simulink model "quad_full_control"  (R2024b)
settings: Solver=ode1  StartTime=0.0  StopTime=inf  FixedStep=0.01  RelTol=1e-3
libraries: slpidlib x4, uavutilslib x1
settings Model: Creator=ercu  LastModifiedBy=ercu

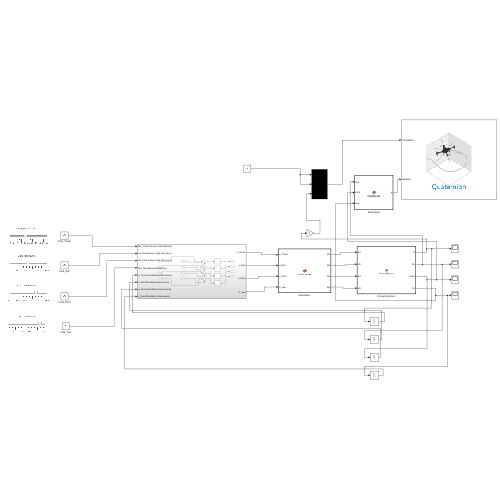
[thumbnail: Simulink's stored preview of the top-level diagram]
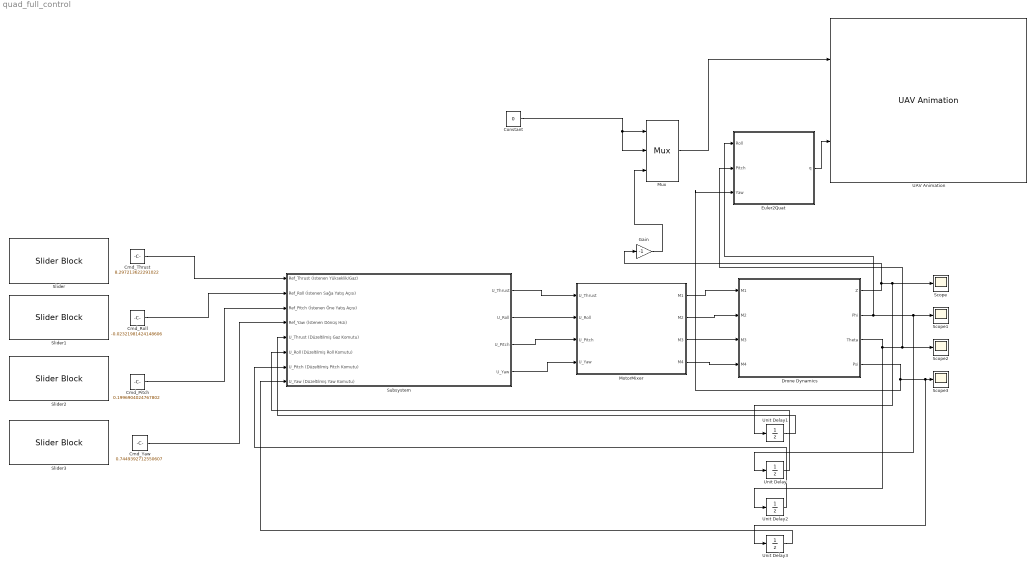
== system quad_full_control ==
  Cmd_Pitch : Constant  Value=0.1996904024767802
  Cmd_Roll : Constant  Value=-0.02321981424148606
  Cmd_Thrust : Constant  Value=8.297213622291022
  Cmd_Yaw : Constant  Value=0.7449392712550607
  Constant : Constant  Value=0
  Drone Dynamics : MATLAB Function  TreatAsAtomicUnit=on
  Euler2Quat : MATLAB Function  TreatAsAtomicUnit=on
  Gain : Gain  Gain=-1
  MotorMixer : MATLAB Function  TreatAsAtomicUnit=on
  Mux : Mux  Inputs=3
  Scope{,1..3} (4 alike) : Scope
  Slider : SliderBlock  ScaleMax=20
  Slider1 : SliderBlock  ScaleMin=-0.5  ScaleMax=0.5
  Slider2 : SliderBlock  ScaleMin=-0.5  ScaleMax=0.5
  Slider3 : SliderBlock  ScaleMin=-1  ScaleMax=1
  Subsystem : Subsystem
  UAV Animation : uavutilslib/UAV Animation  NumUAV=1  DynamicUAVConfig=off  UAVType=Multirotor  UAVSize=1  UAVColor=[1 0 0]  UAVTrajectoryAlpha=1  InertialZDirection=Down  RotationFormat=Quaternion  DrawMarkers=off  SampleTime=-1
  Unit Delay{,1..3} (4 alike) : UnitDelay  SampleTime=-1  HasFrameUpgradeWarning=on
  wires:
  MotorMixer/1(M1) -> Drone Dynamics/1(M1)
  MotorMixer/2(M2) -> Drone Dynamics/2(M2)
  MotorMixer/3(M3) -> Drone Dynamics/3(M3)
  MotorMixer/4(M4) -> Drone Dynamics/4(M4)
  Subsystem/1(U_Thrust) -> MotorMixer/1(U_Thrust)
  Subsystem/2(U_Roll) -> MotorMixer/2(U_Roll)
  Subsystem/3(U_Pitch) -> MotorMixer/3(U_Pitch)
  Subsystem/4(U_Yaw) -> MotorMixer/4(U_Yaw)
  Cmd_Roll/1 -> Subsystem/2(Ref_Roll (İstenen Sağa Yatış Açısı))
  Cmd_Pitch/1 -> Subsystem/3(Ref_Pitch (İstenen Öne Yatış Açısı))
  Cmd_Yaw/1 -> Subsystem/4(Ref_Yaw (İstenen Dönüş Hızı))
  Drone Dynamics/1(Z) -> Gain/1, Unit Delay1/1, Scope/1
  Drone Dynamics/2(Phi) -> Euler2Quat/1(Roll), Unit Delay/1, Scope1/1
  Drone Dynamics/3(Theta) -> Unit Delay2/1, Euler2Quat/2(Pitch), Scope2/1
  Drone Dynamics/4(Psi) -> Euler2Quat/3(Yaw), Unit Delay3/1, Scope3/1
  Unit Delay1/1 -> Subsystem/5(U_Thrust (Düzeltilmiş Gaz Komutu))
  Unit Delay/1 -> Subsystem/6(U_Roll (Düzeltilmiş Roll Komutu))
  Unit Delay2/1 -> Subsystem/7(U_Pitch (Düzeltilmiş Pitch Komutu))
  Unit Delay3/1 -> Subsystem/8(U_Yaw (Düzeltilmiş Yaw Komutu))
  Constant/1 -> Mux/2, Mux/1
  Mux/1 -> UAV Animation/1
  Euler2Quat/1(q) -> UAV Animation/2
  Cmd_Thrust/1 -> Subsystem/1(Ref_Thrust (İstenen Yükseklik/Gaz))
  Gain/1 -> Mux/3

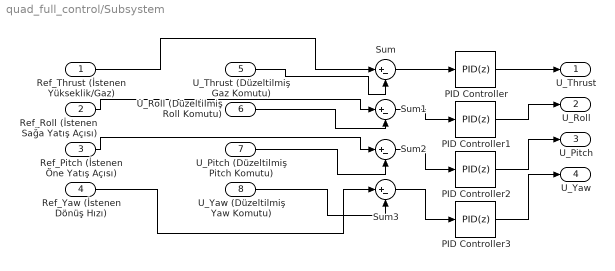
== system quad_full_control/Subsystem ==
  Ref_Thrust (İstenen Yükseklik/Gaz) : Inport
  Ref_Roll (İstenen Sağa Yatış Açısı) : Inport  Port=2
  Ref_Pitch (İstenen Öne Yatış Açısı) : Inport  Port=3
  Ref_Yaw (İstenen Dönüş Hızı) : Inport  Port=4
  U_Thrust (Düzeltilmiş Gaz Komutu) : Inport  Port=5
  U_Roll (Düzeltilmiş Roll Komutu) : Inport  Port=6
  U_Pitch (Düzeltilmiş Pitch Komutu) : Inport  Port=7
  U_Yaw (Düzeltilmiş Yaw Komutu) : Inport  Port=8
  PID Controller : slpidlib/PID Controller  Controller=PID  Form=Parallel  TimeDomain=Discrete-time  UseExternalTs=off  SampleTime=0.01  IntegratorMethod=Forward Euler  FilterMethod=Forward Euler  ControllerParametersSource=internal  P=3  I=1.5  UseKiTs=off  D=2.5  UseExternalDerivativeSource=off  N=100  UseFilter=on  TunerSelectOption=Transfer Function Based (PID Tuner App)  InitialConditionSource=internal  InitialConditionForIntegrator=0  InitialConditionForFilter=0  DifferentiatorICPrevScaledInput=0  ExternalReset=none  TrackingMode=off  Kt=1  LimitOutput=off  SatLimitsSource=internal  UpperSaturationLimit=inf  LowerSaturationLimit=-inf  LinearizeAsGain=on  AntiWindupMode=none  Kb=1  LimitIntegrator=off  UpperIntegratorSaturationLimit=inf  LowerIntegratorSaturationLimit=-inf  POutMin=[]  POutMax=[]  IOutMin=[]  IOutMax=[]  DOutMin=[]  DOutMax=[]  NOutMin=[]  NOutMax=[]  SumOutMin=[]  SumOutMax=[]  SaturationOutMin=[]  SaturationOutMax=[]  PParamMin=[]  PParamMax=[]  IParamMin=[]  IParamMax=[]  DParamMin=[]  DParamMax=[]  NParamMin=[]  NParamMax=[]  KbParamMin=[]  KbParamMax=[]  KtParamMin=[]  KtParamMax=[]  KbOutMin=[]  KbOutMax=[]  KtOutMin=[]  KtOutMax=[]  IntegratorOutMin=[]  IntegratorOutMax=[]  FilterOutMin=[]  FilterOutMax=[]  SumI1OutMin=[]  SumI1OutMax=[]  SumI2OutMin=[]  SumI2OutMax=[]  SumI3OutMin=[]  SumI3OutMax=[]  SumI4OutMin=[]  SumI4OutMax=[]  SumDOutMin=[]  SumDOutMax=[]  DifferentiatorOutMin=[]  DifferentiatorOutMax=[]  FilterDiffOutCoefMin=[]  FilterDiffOutCoefMax=[]  ReciprocalOutMin=[]  ReciprocalOutMax=[]  SumDenOutMin=[]  SumDenOutMax=[]  SumNumOutMin=[]  SumNumOutMax=[]  DivideOutMin=[]  DivideOutMax=[]  UdiffTsProdOutMin=[]  UdiffTsProdOutMax=[]  NTsProdOutMin=[]  NTsProdOutMax=[]  UintegralTsProdOutMin=[]  UintegralTsProdOutMax=[]  UngainTsProdOutMin=[]  UngainTsProdOutMax=[]  ClampingZeroOutDataTypeStr=Inherit: Inherit via back propagation  ClampingZeroOutMin=[]  ClampingZeroOutMax=[]  FilterDenConstantOutDataTypeStr=Inherit: Inherit via back propagation  FilterDenConstantOutMin=[]  FilterDenConstantOutMax=[]  PCopyOutDataTypeStr=Inherit: Inherit via back propagation  PCopyOutMin=[]  PCopyOutMax=[]  NCopyOutDataTypeStr=Inherit: Inherit via back propagation  NCopyOutMin=[]  NCopyOutMax=[]  IntegratorContinuousStateAttributes=''  IntegratorStateMustResolveToSignalObject=off  IntegratorRTWStateStorageClass=Auto  FilterContinuousStateAttributes=''  FilterStateMustResolveToSignalObject=off  FilterRTWStateStorageClass=Auto  ParallelPVariant=InternalParameters  IdealPVariant=Disabled  IVariant=InternalParameters  DVariant=InternalParameters  IntegratorVariant=Discrete  SatVariant=Disabled  AWVariant=Passthrough  PCopyVariant=Disabled  TRVariant=Disabled  FdbkBlocksVariant=Forward  IdealPFdbkVariant=Disabled  SatFdbkVariant=Disabled  DerivativeFilterVariant=ForwardEulerFilter  NVariant=InternalParameters  NCopyVariant=Disabled  FilterICVariant=InternalICsFilter  IntegratorICVariant=InternalICs  ExternalResetVariant=Disabled  TRSumVariant=Passthrough  SumFdbkVariant=Disabled  SumVariant=Sum_PID  TsampFilterVariant=InternalTs  TsampNgainVariant=Passthrough  TsampIntegralVariant=Disabled_SignalSpec  ExternalSaturationOutDataTypeStr=Inherit: Same as second input  DerivativeSourceVariant=ErrorSignal  PreIntVariant=InternalPreInt
  PID Controller1 : slpidlib/PID Controller  Controller=PID  Form=Parallel  TimeDomain=Discrete-time  UseExternalTs=off  SampleTime=0.01  IntegratorMethod=Forward Euler  FilterMethod=Forward Euler  ControllerParametersSource=internal  P=2  I=0  UseKiTs=off  D=0.5  UseExternalDerivativeSource=off  N=100  UseFilter=on  TunerSelectOption=Transfer Function Based (PID Tuner App)  InitialConditionSource=internal  InitialConditionForIntegrator=0  InitialConditionForFilter=0  DifferentiatorICPrevScaledInput=0  ExternalReset=none  TrackingMode=off  Kt=1  LimitOutput=off  SatLimitsSource=internal  UpperSaturationLimit=inf  LowerSaturationLimit=-inf  LinearizeAsGain=on  AntiWindupMode=none  Kb=1  LimitIntegrator=off  UpperIntegratorSaturationLimit=inf  LowerIntegratorSaturationLimit=-inf  POutMin=[]  POutMax=[]  IOutMin=[]  IOutMax=[]  DOutMin=[]  DOutMax=[]  NOutMin=[]  NOutMax=[]  SumOutMin=[]  SumOutMax=[]  SaturationOutMin=[]  SaturationOutMax=[]  PParamMin=[]  PParamMax=[]  IParamMin=[]  IParamMax=[]  DParamMin=[]  DParamMax=[]  NParamMin=[]  NParamMax=[]  KbParamMin=[]  KbParamMax=[]  KtParamMin=[]  KtParamMax=[]  KbOutMin=[]  KbOutMax=[]  KtOutMin=[]  KtOutMax=[]  IntegratorOutMin=[]  IntegratorOutMax=[]  FilterOutMin=[]  FilterOutMax=[]  SumI1OutMin=[]  SumI1OutMax=[]  SumI2OutMin=[]  SumI2OutMax=[]  SumI3OutMin=[]  SumI3OutMax=[]  SumI4OutMin=[]  SumI4OutMax=[]  SumDOutMin=[]  SumDOutMax=[]  DifferentiatorOutMin=[]  DifferentiatorOutMax=[]  FilterDiffOutCoefMin=[]  FilterDiffOutCoefMax=[]  ReciprocalOutMin=[]  ReciprocalOutMax=[]  SumDenOutMin=[]  SumDenOutMax=[]  SumNumOutMin=[]  SumNumOutMax=[]  DivideOutMin=[]  DivideOutMax=[]  UdiffTsProdOutMin=[]  UdiffTsProdOutMax=[]  NTsProdOutMin=[]  NTsProdOutMax=[]  UintegralTsProdOutMin=[]  UintegralTsProdOutMax=[]  UngainTsProdOutMin=[]  UngainTsProdOutMax=[]  ClampingZeroOutDataTypeStr=Inherit: Inherit via back propagation  ClampingZeroOutMin=[]  ClampingZeroOutMax=[]  FilterDenConstantOutDataTypeStr=Inherit: Inherit via back propagation  FilterDenConstantOutMin=[]  FilterDenConstantOutMax=[]  PCopyOutDataTypeStr=Inherit: Inherit via back propagation  PCopyOutMin=[]  PCopyOutMax=[]  NCopyOutDataTypeStr=Inherit: Inherit via back propagation  NCopyOutMin=[]  NCopyOutMax=[]  IntegratorContinuousStateAttributes=''  IntegratorStateMustResolveToSignalObject=off  IntegratorRTWStateStorageClass=Auto  FilterContinuousStateAttributes=''  FilterStateMustResolveToSignalObject=off  FilterRTWStateStorageClass=Auto  ParallelPVariant=InternalParameters  IdealPVariant=Disabled  IVariant=InternalParameters  DVariant=InternalParameters  IntegratorVariant=Discrete  SatVariant=Disabled  AWVariant=Passthrough  PCopyVariant=Disabled  TRVariant=Disabled  FdbkBlocksVariant=Forward  IdealPFdbkVariant=Disabled  SatFdbkVariant=Disabled  DerivativeFilterVariant=ForwardEulerFilter  NVariant=InternalParameters  NCopyVariant=Disabled  FilterICVariant=InternalICsFilter  IntegratorICVariant=InternalICs  ExternalResetVariant=Disabled  TRSumVariant=Passthrough  SumFdbkVariant=Disabled  SumVariant=Sum_PID  TsampFilterVariant=InternalTs  TsampNgainVariant=Passthrough  TsampIntegralVariant=Disabled_SignalSpec  ExternalSaturationOutDataTypeStr=Inherit: Same as second input  DerivativeSourceVariant=ErrorSignal  PreIntVariant=InternalPreInt
  PID Controller2 : slpidlib/PID Controller  Controller=PID  Form=Parallel  TimeDomain=Discrete-time  UseExternalTs=off  SampleTime=0.01  IntegratorMethod=Forward Euler  FilterMethod=Forward Euler  ControllerParametersSource=internal  P=2  I=0  UseKiTs=off  D=0.5  UseExternalDerivativeSource=off  N=100  UseFilter=on  TunerSelectOption=Transfer Function Based (PID Tuner App)  InitialConditionSource=internal  InitialConditionForIntegrator=0  InitialConditionForFilter=0  DifferentiatorICPrevScaledInput=0  ExternalReset=none  TrackingMode=off  Kt=1  LimitOutput=off  SatLimitsSource=internal  UpperSaturationLimit=inf  LowerSaturationLimit=-inf  LinearizeAsGain=on  AntiWindupMode=none  Kb=1  LimitIntegrator=off  UpperIntegratorSaturationLimit=inf  LowerIntegratorSaturationLimit=-inf  POutMin=[]  POutMax=[]  IOutMin=[]  IOutMax=[]  DOutMin=[]  DOutMax=[]  NOutMin=[]  NOutMax=[]  SumOutMin=[]  SumOutMax=[]  SaturationOutMin=[]  SaturationOutMax=[]  PParamMin=[]  PParamMax=[]  IParamMin=[]  IParamMax=[]  DParamMin=[]  DParamMax=[]  NParamMin=[]  NParamMax=[]  KbParamMin=[]  KbParamMax=[]  KtParamMin=[]  KtParamMax=[]  KbOutMin=[]  KbOutMax=[]  KtOutMin=[]  KtOutMax=[]  IntegratorOutMin=[]  IntegratorOutMax=[]  FilterOutMin=[]  FilterOutMax=[]  SumI1OutMin=[]  SumI1OutMax=[]  SumI2OutMin=[]  SumI2OutMax=[]  SumI3OutMin=[]  SumI3OutMax=[]  SumI4OutMin=[]  SumI4OutMax=[]  SumDOutMin=[]  SumDOutMax=[]  DifferentiatorOutMin=[]  DifferentiatorOutMax=[]  FilterDiffOutCoefMin=[]  FilterDiffOutCoefMax=[]  ReciprocalOutMin=[]  ReciprocalOutMax=[]  SumDenOutMin=[]  SumDenOutMax=[]  SumNumOutMin=[]  SumNumOutMax=[]  DivideOutMin=[]  DivideOutMax=[]  UdiffTsProdOutMin=[]  UdiffTsProdOutMax=[]  NTsProdOutMin=[]  NTsProdOutMax=[]  UintegralTsProdOutMin=[]  UintegralTsProdOutMax=[]  UngainTsProdOutMin=[]  UngainTsProdOutMax=[]  ClampingZeroOutDataTypeStr=Inherit: Inherit via back propagation  ClampingZeroOutMin=[]  ClampingZeroOutMax=[]  FilterDenConstantOutDataTypeStr=Inherit: Inherit via back propagation  FilterDenConstantOutMin=[]  FilterDenConstantOutMax=[]  PCopyOutDataTypeStr=Inherit: Inherit via back propagation  PCopyOutMin=[]  PCopyOutMax=[]  NCopyOutDataTypeStr=Inherit: Inherit via back propagation  NCopyOutMin=[]  NCopyOutMax=[]  IntegratorContinuousStateAttributes=''  IntegratorStateMustResolveToSignalObject=off  IntegratorRTWStateStorageClass=Auto  FilterContinuousStateAttributes=''  FilterStateMustResolveToSignalObject=off  FilterRTWStateStorageClass=Auto  ParallelPVariant=InternalParameters  IdealPVariant=Disabled  IVariant=InternalParameters  DVariant=InternalParameters  IntegratorVariant=Discrete  SatVariant=Disabled  AWVariant=Passthrough  PCopyVariant=Disabled  TRVariant=Disabled  FdbkBlocksVariant=Forward  IdealPFdbkVariant=Disabled  SatFdbkVariant=Disabled  DerivativeFilterVariant=ForwardEulerFilter  NVariant=InternalParameters  NCopyVariant=Disabled  FilterICVariant=InternalICsFilter  IntegratorICVariant=InternalICs  ExternalResetVariant=Disabled  TRSumVariant=Passthrough  SumFdbkVariant=Disabled  SumVariant=Sum_PID  TsampFilterVariant=InternalTs  TsampNgainVariant=Passthrough  TsampIntegralVariant=Disabled_SignalSpec  ExternalSaturationOutDataTypeStr=Inherit: Same as second input  DerivativeSourceVariant=ErrorSignal  PreIntVariant=InternalPreInt
  PID Controller3 : slpidlib/PID Controller  Controller=PID  Form=Parallel  TimeDomain=Discrete-time  UseExternalTs=off  SampleTime=0.01  IntegratorMethod=Forward Euler  FilterMethod=Forward Euler  ControllerParametersSource=internal  P=4  I=0.5  UseKiTs=off  D=0  UseExternalDerivativeSource=off  N=100  UseFilter=on  TunerSelectOption=Transfer Function Based (PID Tuner App)  InitialConditionSource=internal  InitialConditionForIntegrator=0  InitialConditionForFilter=0  DifferentiatorICPrevScaledInput=0  ExternalReset=none  TrackingMode=off  Kt=1  LimitOutput=off  SatLimitsSource=internal  UpperSaturationLimit=inf  LowerSaturationLimit=-inf  LinearizeAsGain=on  AntiWindupMode=none  Kb=1  LimitIntegrator=off  UpperIntegratorSaturationLimit=inf  LowerIntegratorSaturationLimit=-inf  POutMin=[]  POutMax=[]  IOutMin=[]  IOutMax=[]  DOutMin=[]  DOutMax=[]  NOutMin=[]  NOutMax=[]  SumOutMin=[]  SumOutMax=[]  SaturationOutMin=[]  SaturationOutMax=[]  PParamMin=[]  PParamMax=[]  IParamMin=[]  IParamMax=[]  DParamMin=[]  DParamMax=[]  NParamMin=[]  NParamMax=[]  KbParamMin=[]  KbParamMax=[]  KtParamMin=[]  KtParamMax=[]  KbOutMin=[]  KbOutMax=[]  KtOutMin=[]  KtOutMax=[]  IntegratorOutMin=[]  IntegratorOutMax=[]  FilterOutMin=[]  FilterOutMax=[]  SumI1OutMin=[]  SumI1OutMax=[]  SumI2OutMin=[]  SumI2OutMax=[]  SumI3OutMin=[]  SumI3OutMax=[]  SumI4OutMin=[]  SumI4OutMax=[]  SumDOutMin=[]  SumDOutMax=[]  DifferentiatorOutMin=[]  DifferentiatorOutMax=[]  FilterDiffOutCoefMin=[]  FilterDiffOutCoefMax=[]  ReciprocalOutMin=[]  ReciprocalOutMax=[]  SumDenOutMin=[]  SumDenOutMax=[]  SumNumOutMin=[]  SumNumOutMax=[]  DivideOutMin=[]  DivideOutMax=[]  UdiffTsProdOutMin=[]  UdiffTsProdOutMax=[]  NTsProdOutMin=[]  NTsProdOutMax=[]  UintegralTsProdOutMin=[]  UintegralTsProdOutMax=[]  UngainTsProdOutMin=[]  UngainTsProdOutMax=[]  ClampingZeroOutDataTypeStr=Inherit: Inherit via back propagation  ClampingZeroOutMin=[]  ClampingZeroOutMax=[]  FilterDenConstantOutDataTypeStr=Inherit: Inherit via back propagation  FilterDenConstantOutMin=[]  FilterDenConstantOutMax=[]  PCopyOutDataTypeStr=Inherit: Inherit via back propagation  PCopyOutMin=[]  PCopyOutMax=[]  NCopyOutDataTypeStr=Inherit: Inherit via back propagation  NCopyOutMin=[]  NCopyOutMax=[]  IntegratorContinuousStateAttributes=''  IntegratorStateMustResolveToSignalObject=off  IntegratorRTWStateStorageClass=Auto  FilterContinuousStateAttributes=''  FilterStateMustResolveToSignalObject=off  FilterRTWStateStorageClass=Auto  ParallelPVariant=InternalParameters  IdealPVariant=Disabled  IVariant=InternalParameters  DVariant=InternalParameters  IntegratorVariant=Discrete  SatVariant=Disabled  AWVariant=Passthrough  PCopyVariant=Disabled  TRVariant=Disabled  FdbkBlocksVariant=Forward  IdealPFdbkVariant=Disabled  SatFdbkVariant=Disabled  DerivativeFilterVariant=ForwardEulerFilter  NVariant=InternalParameters  NCopyVariant=Disabled  FilterICVariant=InternalICsFilter  IntegratorICVariant=InternalICs  ExternalResetVariant=Disabled  TRSumVariant=Passthrough  SumFdbkVariant=Disabled  SumVariant=Sum_PID  TsampFilterVariant=InternalTs  TsampNgainVariant=Passthrough  TsampIntegralVariant=Disabled_SignalSpec  ExternalSaturationOutDataTypeStr=Inherit: Same as second input  DerivativeSourceVariant=ErrorSignal  PreIntVariant=InternalPreInt
  Sum{,1..3} (4 alike) : Sum  Inputs=|+-
  U_Thrust : Outport
  U_Roll : Outport  Port=2
  U_Pitch : Outport  Port=3
  U_Yaw : Outport  Port=4
  wires:
  Ref_Thrust (İstenen Yükseklik/Gaz)/1 -> Sum/1
  Ref_Roll (İstenen Sağa Yatış Açısı)/1 -> Sum1/1
  Ref_Pitch (İstenen Öne Yatış Açısı)/1 -> Sum2/1
  Ref_Yaw (İstenen Dönüş Hızı)/1 -> Sum3/1
  U_Pitch (Düzeltilmiş Pitch Komutu)/1 -> Sum2/2
  U_Roll (Düzeltilmiş Roll Komutu)/1 -> Sum1/2
  U_Thrust (Düzeltilmiş Gaz Komutu)/1 -> Sum/2
  Sum/1 -> PID Controller/1
  Sum1/1 -> PID Controller1/1
  Sum2/1 -> PID Controller2/1
  Sum3/1 -> PID Controller3/1
  PID Controller/1 -> U_Thrust/1
  PID Controller1/1 -> U_Roll/1
  PID Controller2/1 -> U_Pitch/1
  PID Controller3/1 -> U_Yaw/1
  U_Yaw (Düzeltilmiş Yaw Komutu)/1 -> Sum3/2

== matlab function quad_full_control/Drone Dynamics ==
  data: M1 input; Z output; M2 input; M3 input; M4 input; Phi output; Theta output; Psi output
function [Z, Phi, Theta, Psi] = DronePhysics(M1, M2, M3, M4)
    % Drone Fizigi - ACI KONTROL MODU (Angle Control)
    % Z: Yukseklik, Phi: Roll, Theta: Pitch, Psi: Yaw
    
    persistent p_Z p_Phi p_Theta p_Psi v_Z v_Phi v_Theta v_Psi
    
    if isempty(p_Z)
        p_Z=0; p_Phi=0; p_Theta=0; p_Psi=0;
        v_Z=0; v_Phi=0; v_Theta=0; v_Psi=0;
    end
    
    dt = 0.01; 
    m = 1.2;   
    g = 9.81;
    Ixx = 0.01; Iyy = 0.01; Izz = 0.02; 
    
    % Kuvvetler
    F_total = M1 + M2 + M3 + M4;
    Tau_Roll = (M2 + M3) - (M1 + M4); 
    Tau_Pitch = (M1 + M3) - (M2 + M4); 
    Tau_Yaw = (M1 + M2) - (M3 + M4); 
    
    % --- SURTUNME (DAMPING) ---
    % Dronun donusunu yavaslatmak icin sart
    b_rot = 0.5; 
    
    % 1. Z Ekseni
    acc_Z = (F_total / m) - g;
    v_Z = v_Z + acc_Z * dt;
    p_Z = p_Z + v_Z * dt;
    if p_Z < 0; p_Z = 0; v_Z = 0; end 
    
    % 2. Acisal Hareket (Surtunmeli)
    alpha_Roll = (Tau_Roll - (v_Phi * b_rot)) / Ixx;
    alpha_Pitch = (Tau_Pitch - (v_Theta * b_rot)) / Iyy;
    alpha_Yaw = (Tau_Yaw - (v_Psi * b_rot)) / Izz;
    
    % Integrasyon
    v_Phi = v_Phi + alpha_Roll * dt;
    p_Phi = p_Phi + v_Phi * dt;
    
    v_Theta = v_Theta + alpha_Pitch * dt;
    p_Theta = p_Theta + v_Theta * dt;
    
    v_Psi = v_Psi + alpha_Yaw * dt;
    p_Psi = p_Psi + v_Psi * dt;
    
    % Cikislar (Sadece Acilar)
    Z = p_Z;
    Phi = p_Phi;
    Theta = p_Theta;
    Psi = p_Psi; 
end

== matlab function quad_full_control/MotorMixer ==
  data: U_Thrust input; M1 output; U_Roll input; U_Pitch input; U_Yaw input; M2 output; M3 output; M4 output
function [M1, M2, M3, M4] = MotorMixer(U_Thrust, U_Roll, U_Pitch, U_Yaw)
    % Quadcopter X Config Motor Mixing Algorithm
    % M1: Sag On (CCW), M2: Sol Arka (CCW) -> Tersi yonler
    % M3: Sol On (CW),  M4: Sag Arka (CW)
    
    % Temel Mantik:
    % Roll sag istiyorsa -> Sol motorlari artir, Sag motorlari azalt.
    % Pitch on istiyorsa -> Arka motorlari artir, On motorlari azalt.
    
    % Mixing Matrix
    M1 = U_Thrust - U_Roll + U_Pitch + U_Yaw; % Sag On
    M2 = U_Thrust + U_Roll - U_Pitch + U_Yaw; % Sol Arka
    M3 = U_Thrust + U_Roll + U_Pitch - U_Yaw; % Sol On
    M4 = U_Thrust - U_Roll - U_Pitch - U_Yaw; % Sag Arka
    
    % Motor Limitleri (Saturation)
    % Motorlar eksi donemez, max 30N uretebilir
    M1 = min(max(M1, 0), 30);
    M2 = min(max(M2, 0), 30);
    M3 = min(max(M3, 0), 30);
    M4 = min(max(M4, 0), 30);
end

== matlab function quad_full_control/Euler2Quat ==
  data: Roll input; q output; Pitch input; Yaw input
function q = Euler2Quat(Roll, Pitch, Yaw)
    % Simulink Code Gen uyumlu Manuel Donusum
    % Euler ZYX Siralamasi (Yaw -> Pitch -> Roll)
    
    % Yari acilarin cos ve sin degerleri
    c1 = cos(Yaw / 2);
    s1 = sin(Yaw / 2);
    c2 = cos(Pitch / 2);
    s2 = sin(Pitch / 2);
    c3 = cos(Roll / 2);
    s3 = sin(Roll / 2);

    % Quaternion bilesenleri (w, x, y, z)
    w = c1 * c2 * c3 + s1 * s2 * s3;
    x = c1 * c2 * s3 - s1 * s2 * c3;
    y = c1 * s2 * c3 + s1 * c2 * s3;
    z = s1 * c2 * c3 - c1 * s2 * s3;

    % Cikis vektoru (1x4)
    q = [w, x, y, z];
end
